simulink model "GPS_IOT_new"  (R2024b)
settings: Solver=VariableStepAuto  StartTime=0.0  StopTime=60  RelTol=1e-3
StopFcn:
  | try
  |     if evalin('base', 'exist(''latitude'', ''var'')') && evalin('base', 'exist(''longitude'', ''var'')')
  |         latitude = evalin('base', 'latitude');
  |         longitude = evalin('base', 'longitude');
  |         status = evalin('base', 'status');
  |         distance = evalin('base', 'distance');
  | 
  |         % Ensure latitude & longitude are scalars before sending to Firebase
  |         if isscalar(latitude) && isscalar(longitude)
  |             send_to_firebase(latitude, longitude, status, distance);
  |         else
  |             disp('❗ Latitude or Longitude are arrays, expected scalars.');
  |         end
  |     else
  |         disp('❗ Latitude or Longitude not found in workspace.');
  |     end
  | catch ME
  |     disp('❌ Error in StopFcn while sending to Firebase:');
  |     disp(getReport(ME));
  | end
settings Model: Creator=NANDAN  LastModifiedBy=NANDAN

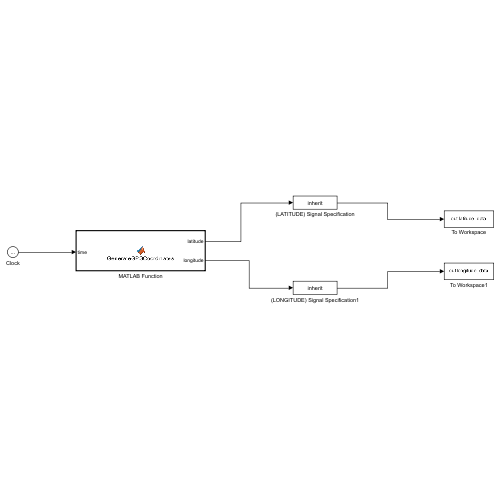
[thumbnail: Simulink's stored preview of the top-level diagram]
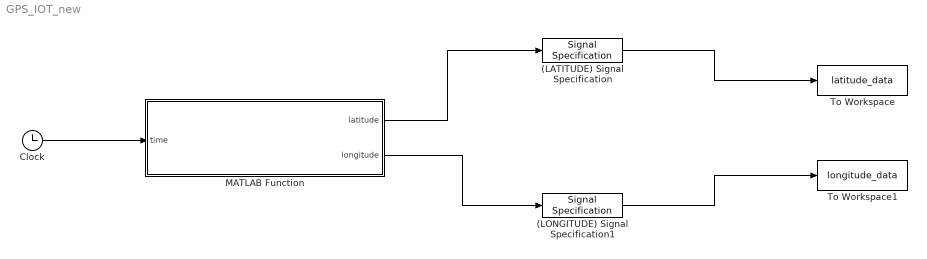
== system GPS_IOT_new ==
  (LATITUDE) Signal Specification : SignalSpecification
  (LONGITUDE) Signal Specification1 : SignalSpecification
  Clock : Clock
  MATLAB Function : MATLAB Function  TreatAsAtomicUnit=on
  To Workspace : ToWorkspace  VariableName=latitude_data  SampleTime=-1
  To Workspace1 : ToWorkspace  VariableName=longitude_data  SampleTime=-1
  wires:
  Clock/1 -> MATLAB Function/1(time)
  MATLAB Function/1(latitude) -> (LATITUDE) Signal Specification/1
  MATLAB Function/2(longitude) -> (LONGITUDE) Signal Specification1/1
  (LATITUDE) Signal Specification/1 -> To Workspace/1
  (LONGITUDE) Signal Specification1/1 -> To Workspace1/1

== matlab function GPS_IOT_new/MATLAB Function ==
  data: time input; latitude output; longitude output
function [latitude, longitude] = GenerateGPSCoordinates(time)
%#codegen

% Explicitly define outputs before assignment
latitude = 0; 
longitude = 0;

% ✅ Permanent Base Location (Modify this manually if needed)
persistent printedBaseLocation;
baseLat = 12.9746;  
baseLon = 77.5988;  

if isempty(printedBaseLocation)
    printedBaseLocation = true;
    disp("=== Permanent Base Location ===");
    disp("Latitude: " + num2str(baseLat) + " | Longitude: " + num2str(baseLon));
end

% ✅ Moving Location (Modify manually for testing geofencing behavior)
movingLat = 12.9749;  % Adjust manually to test geofence status
movingLon = 77.5987;  % Adjust manually to test geofence status

% ✅ Haversine Formula to Calculate Distance Dynamically
R = 6371; % Radius of Earth in kilometers
dLat = deg2rad(movingLat - baseLat);
dLon = deg2rad(movingLon - baseLon);
a = sin(dLat/2)^2 + cos(deg2rad(baseLat)) * cos(deg2rad(movingLat)) * sin(dLon/2)^2;
c = 2 * atan2(sqrt(a), sqrt(1-a));
distance = R * c * 1000; % Convert km to meters

% ✅ Fix `round(distance,2)` → Use `fix()`
fixedDistance = fix(distance * 100) / 100;

% ✅ Geofence Check (Inside or Outside 50m)
if fixedDistance <= 50
    status = "INSIDE Geofence";
else
    status = "OUTSIDE Geofence";
end

% ✅ Store values for Firebase update
assignin('base', 'latitude', movingLat);
assignin('base', 'longitude', movingLon);
assignin('base', 'status', status);
assignin('base', 'distance', fixedDistance);
end
